simulink model "Gravity_gradient"  (R2021b)
settings: Solver=VariableStepAuto  StartTime=0.0  StopTime=SimTime  RelTol=1e-3
settings Model: Creator=adity  LastModifiedBy=adity

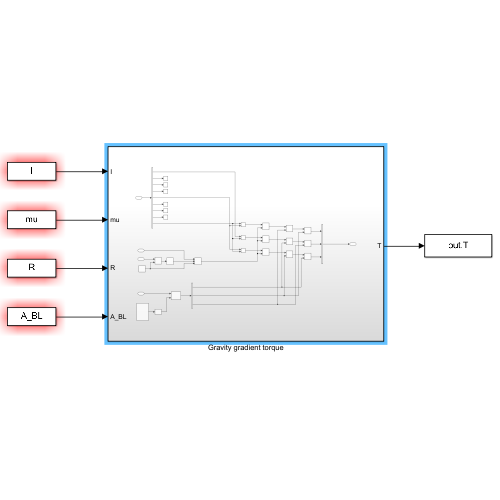
[thumbnail: Simulink's stored preview of the top-level diagram]
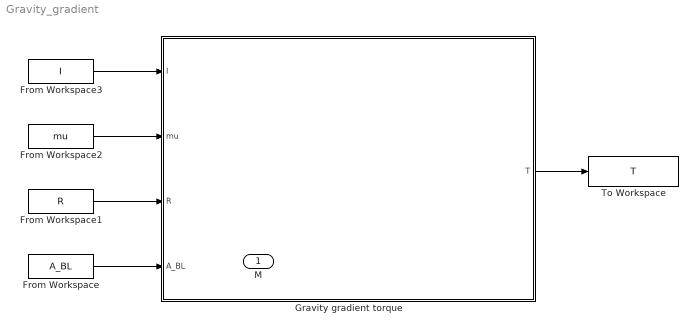
== system Gravity_gradient ==
  From Workspace : FromWorkspace  VariableName=A_BL
  From Workspace1 : FromWorkspace  VariableName=R
  From Workspace2 : FromWorkspace  VariableName=mu
  From Workspace3 : FromWorkspace  VariableName=I
  Gravity gradient torque : Subsystem
  To Workspace : ToWorkspace  VariableName=T  SaveFormat=Timeseries  SampleTime=-1
  M : Outport
  wires:
  From Workspace3/1 -> Gravity gradient torque/1(I)
  From Workspace2/1 -> Gravity gradient torque/2(mu)
  From Workspace1/1 -> Gravity gradient torque/3(R)
  From Workspace/1 -> Gravity gradient torque/4(A_BL)
  Gravity gradient torque/1(T) -> To Workspace/1

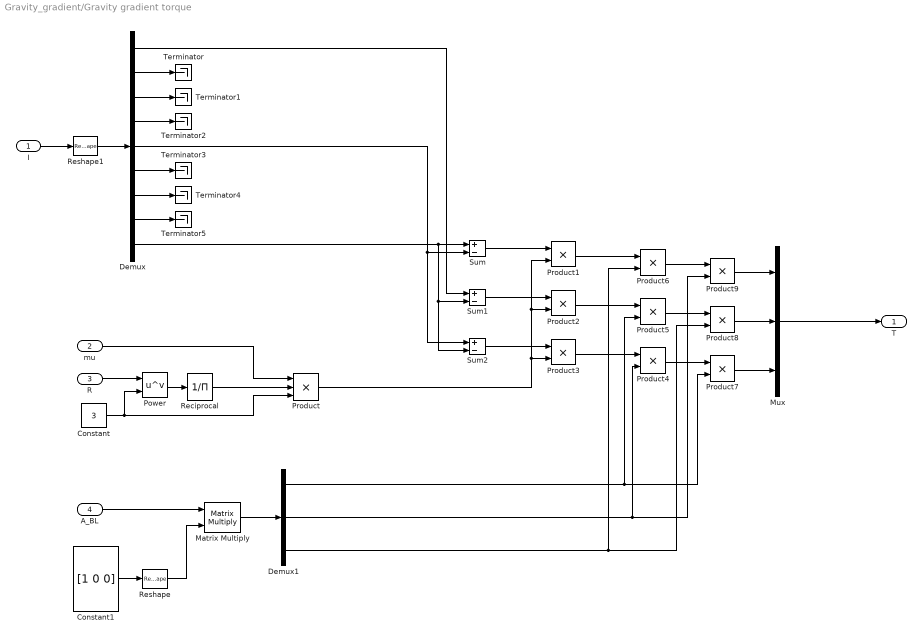
== system Gravity_gradient/Gravity gradient torque ==
  I : Inport
  mu : Inport  Port=2
  R : Inport  Port=3
  A_BL : Inport  Port=4
  Constant : Constant  Value=3
  Constant1 : Constant  Value=[1 0 0]
  Demux : Demux  Outputs=9
  Demux1 : Demux  Outputs=3
  Matrix Multiply : Product  Multiplication=Matrix(*)
  Mux : Mux  Inputs=3
  Power : Math  Operator=pow  SaturateOnIntegerOverflow=on
  Product : Product  Inputs=3
  Product{1..9} (9 alike) : Product
  Reciprocal : Product  Inputs=/
  Reshape : Reshape  OutputDimensionality=Column vector (2-D)
  Reshape1 : Reshape  OutputDimensionality=Column vector (2-D)
  Sum : Sum  Inputs=+-
  Sum1 : Sum  Inputs=+-
  Sum2 : Sum  Inputs=+-
  Terminator{,1..5} (6 alike) : Terminator
  T : Outport
  wires:
  Demux/4 -> Terminator2/1
  Product/1 -> Product3/2, Product1/2, Product2/2
  Constant/1 -> Product/3, Power/2
  Demux1/1 -> Product5/2, Product7/2
  Demux/2 -> Terminator/1
  Product6/1 -> Product9/1
  Sum/1 -> Product1/1
  Product1/1 -> Product6/1
  Demux/7 -> Terminator4/1
  Demux1/3 -> Product6/2, Product8/2
  Power/1 -> Reciprocal/1
  Demux/1 -> Sum1/1
  Product5/1 -> Product8/1
  Demux/3 -> Terminator1/1
  I/1 -> Reshape1/1
  Matrix Multiply/1 -> Demux1/1
  Demux/9 -> Sum2/2, Sum1/2, Sum/1
  Constant1/1 -> Reshape/1
  Sum1/1 -> Product2/1
  Sum2/1 -> Product3/1
  Product7/1 -> Mux/3
  Mux/1 -> T/1
  mu/1 -> Product/1
  R/1 -> Power/1
  Demux/5 -> Sum/2, Sum2/1
  Reciprocal/1 -> Product/2
  Demux/8 -> Terminator5/1
  A_BL/1 -> Matrix Multiply/1
  Product4/1 -> Product7/1
  Product8/1 -> Mux/2
  Demux/6 -> Terminator3/1
  Demux1/2 -> Product4/2, Product9/2
  Product2/1 -> Product5/1
  Product9/1 -> Mux/1
  Product3/1 -> Product4/1
  Reshape/1 -> Matrix Multiply/2
  Reshape1/1 -> Demux/1
